simulink model "robot_model"  (R2018b)
settings: Solver=ode15s  StartTime=0.0  StopTime=26  RelTol=1e-3  EnableMultiTasking=on
values from neighbouring files (symbols this model uses):
  FLC1 = readfis('FLC1')    [start.m]
  fs = 100    [start.m]
libraries: simulink_extras x4, fuzblock x3, simulink x2
settings Model: Creator=Akos  LastModifiedBy=akos
settings DataIOCC: LimitDataPoints=on  SaveFormat=Array
settings OptimizationCC: LifeSpan=inf
settings DebuggingCC: SFUnexpectedBacktrackingDiag=warning  SFNoUnconditionalDefaultTransitionDiag=warning  SFExecutionAtInitializationDiag=none
settings HardwareCC: ProdBitPerPointer=32  ProdBitPerSizeT=32  ProdBitPerPtrDiffT=32  ProdLargestAtomicFloat=None  ProdIntDivRoundTo=Undefined  ProdEndianess=Unspecified  ProdWordSize=32  ProdHWDeviceType=32-bit Generic
settings ModelReferenceCC: PropagateSignalLabelsOutOfModel=off
settings SFSimCC: SimUseLocalCustomCode=off
settings RTWCC: RTWUseLocalCustomCode=off
settings CodeAppCC: StateflowObjectComments=on
settings GRTTargetCC: TargetLangStandard=C89/C90 (ANSI)  GeneratePreprocessorConditionals=Disable all
settings ConfigComp: CovMetricSettings=dw  CovHtmlReporting=on  CovSaveCumulativeToWorkspaceVar=on  CovSaveSingleToWorkspaceVar=on  CovExternalEMLEnable=off

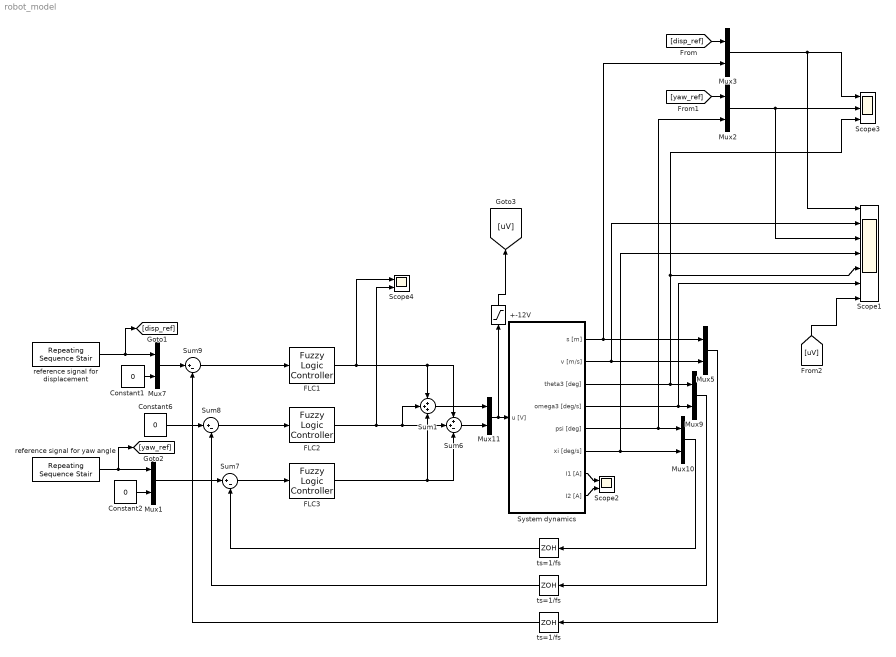
== system robot_model ==
  +-12V : Saturate  UpperLimit=12  LowerLimit=-12
  Constant1 : Constant  Value=0
  Constant2 : Constant  Value=0
  Constant6 : Constant  Value=0
  FLC1 : fuzblock/Fuzzy Logic  Controller  FIS=[FLC1]  OutputSampleNumber=101  DataType=double  FuzzifiedInputs=off  RuleFiringStrengths=off  RuleOutputs=off  AggregatedOutputs=off  SimulateUsing=Interpreted execution  OutOfRangeInputValueMessage=warning  NoRuleFiredMessage=warning  EmptyOutputFuzzySetMessage=warning
  FLC2 : fuzblock/Fuzzy Logic  Controller  FIS=FLC2  OutputSampleNumber=101  DataType=double  FuzzifiedInputs=off  RuleFiringStrengths=off  RuleOutputs=off  AggregatedOutputs=off  SimulateUsing=Interpreted execution  OutOfRangeInputValueMessage=warning  NoRuleFiredMessage=warning  EmptyOutputFuzzySetMessage=warning
  FLC3 : fuzblock/Fuzzy Logic  Controller  FIS=FLC3  OutputSampleNumber=101  DataType=double  FuzzifiedInputs=off  RuleFiringStrengths=off  RuleOutputs=off  AggregatedOutputs=off  SimulateUsing=Interpreted execution  OutOfRangeInputValueMessage=warning  NoRuleFiredMessage=warning  EmptyOutputFuzzySetMessage=warning
  Mux{1..3,5,7,9..11} (8 alike) : Mux  Inputs=2
  Scope1 : Scope  NumInputPorts=7
  Scope2 : Scope  NumInputPorts=2
  Scope3 : Scope  NumInputPorts=3
  Scope4 : Scope  NumInputPorts=2
  Sum1 : Sum  Inputs=+++
  Sum6 : Sum  Inputs=++-
  Sum7 : Sum  Inputs=|+-  SampleTime=1/100
  Sum8 : Sum  Inputs=|+-  SampleTime=1/100
  Sum9 : Sum  Inputs=|+-  SampleTime=1/100
  System dynamics : Subsystem
  reference signal for displacement : simulink/Sources/Repeating Sequence Stair  OutValues=[0 0.1698 0.1698 0.03255 0.03255 -0.1148 0].'  tsamp=4  OutMin=[]  OutMax=[]  OutDataTypeStr=double  OutputDataTypeScalingMode=double  OutDataType=fixdt(0,8)  ConRadixGroup=Best Precision: Vector-wise  OutScaling=2^-12
  reference signal for yaw angle : simulink/Sources/Repeating Sequence Stair  OutValues=[0 0 59.98 59.98 -16.04 -16.04 0].'  tsamp=4  OutMin=[]  OutMax=[]  OutDataTypeStr=double  OutputDataTypeScalingMode=double  OutDataType=fixdt(0,8)  ConRadixGroup=Best Precision: Vector-wise  OutScaling=2^-12
  "ts=1/fs " : ZeroOrderHold  SampleTime=1/fs
  "ts=1/fs  " : ZeroOrderHold  SampleTime=1/fs
  "ts=1/fs   " : ZeroOrderHold  SampleTime=1/fs
  wires:
  System dynamics/7(I1 [A]) -> Scope2/1
  System dynamics/8(I2 [A]) -> Scope2/2
  System dynamics/2(v [m/s]) -> Scope1/2, Mux5/2
  System dynamics/4(omega3 [deg/s]) -> Scope1/6, Mux9/2
  System dynamics/5(psi [deg]) -> Mux10/1, Mux2/2
  System dynamics/6(xi [deg/s]) -> Scope1/4, Mux10/2
  Mux10/1 -> "ts=1/fs "/1
  Mux9/1 -> "ts=1/fs  "/1
  Mux5/1 -> "ts=1/fs   "/1
  Sum7/1 -> FLC3/1
  "ts=1/fs "/1 -> Sum7/2
  "ts=1/fs  "/1 -> Sum8/2
  "ts=1/fs   "/1 -> Sum9/2
  Sum6/1 -> Mux11/2
  Sum1/1 -> Mux11/1
  Mux11/1 -> +-12V/1, System dynamics/1(u [V])
  Mux7/1 -> Sum9/1
  Constant6/1 -> Sum8/1
  Mux1/1 -> Sum7/1
  System dynamics/3(theta3 [deg]) -> Scope1/5, Scope3/3, Mux9/1
  FLC1/1 -> Scope4/1, Sum1/1, Sum6/1
  FLC2/1 -> Scope4/2, Sum1/2, Sum6/2
  System dynamics/1(s [m]) -> Mux5/1, Mux3/2
  reference signal for displacement/1 -> [disp_ref], Mux7/1
  Constant1/1 -> Mux7/2
  Mux3/1 -> Scope1/1, Scope3/1
  Sum9/1 -> FLC1/1
  Sum8/1 -> FLC2/1
  [disp_ref] -> Mux3/1
  Constant2/1 -> Mux1/2
  [yaw_ref] -> Mux2/1
  reference signal for yaw angle/1 -> [yaw_ref], Mux1/1
  FLC3/1 -> Sum6/3, Sum1/3
  Mux2/1 -> Scope1/3, Scope3/2
  [uV] -> Scope1/7
  +-12V/1 -> [uV]

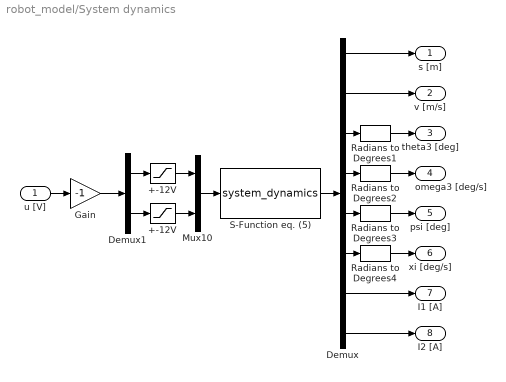
== system robot_model/System dynamics ==
  u [V] : Inport
  +-12V : Saturate  UpperLimit=12  LowerLimit=-12
  "+-12V " : Saturate  UpperLimit=12  LowerLimit=-12
  Demux : Demux  Outputs=8
  Demux1 : Demux  Outputs=2
  Gain : Gain  Gain=-1
  Mux10 : Mux  Inputs=2
  Radians to Degrees{1..4} (4 alike) : simulink_extras/Transformations/Radians to Degrees
  S-Function eq. (5) : S-Function  FunctionName=system_dynamics  SFunctionDeploymentMode=off  EnableBusSupport=off
  s [m] : Outport
  v [m/s] : Outport  Port=2
  theta3 [deg] : Outport  Port=3
  omega3 [deg/s] : Outport  Port=4
  psi [deg] : Outport  Port=5
  xi [deg/s] : Outport  Port=6
  I1 [A] : Outport  Port=7
  I2 [A] : Outport  Port=8
  wires:
  Demux/2 -> v [m/s]/1
  Demux/1 -> s [m]/1
  Demux/3 -> Radians to Degrees1/1
  Demux/7 -> I1 [A]/1
  Demux/8 -> I2 [A]/1
  Mux10/1 -> S-Function eq. (5)/1
  S-Function eq. (5)/1 -> Demux/1
  Demux/6 -> Radians to Degrees4/1
  Demux/5 -> Radians to Degrees3/1
  Demux/4 -> Radians to Degrees2/1
  +-12V/1 -> Mux10/1
  "+-12V "/1 -> Mux10/2
  Radians to Degrees1/1 -> theta3 [deg]/1
  Radians to Degrees2/1 -> omega3 [deg/s]/1
  Radians to Degrees3/1 -> psi [deg]/1
  Radians to Degrees4/1 -> xi [deg/s]/1
  u [V]/1 -> Gain/1
  Demux1/1 -> +-12V/1
  Demux1/2 -> "+-12V "/1
  Gain/1 -> Demux1/1
